simulink model "MEEN432_Project3_start"  (R2024b)
settings: Solver=VariableStepAuto  StartTime=0.0  StopTime=344  RelTol=1e-3
values from neighbouring files (symbols this model uses):
  eff = 0.9    [Project3_init.m]
  epa = urban_epa    [Project3_init.m]
  F_drag = 0    [Project3_init.m]
  G = 100    [Project3_init.m]
  I = 1600    [Project3_init.m]
  I_w = 0    [Project3_init.m]
  input_gear_inertia = 0.1    [Project3_init.m]
  m = 1000    [Project3_init.m]
  output_gear_inertia = 0.001    [Project3_init.m]
  r = 0.3    [Project3_init.m]
  tau_l = 1    [Project3_init.m]
  time = urban_time    [Project3_init.m]
  Tm_max = 350    [Project3_init.m]
libraries: slpidlib x1
settings Model: Creator=flare  LastModifiedBy=jpalm
settings RTWCC: GPUComputeCapability=3.5

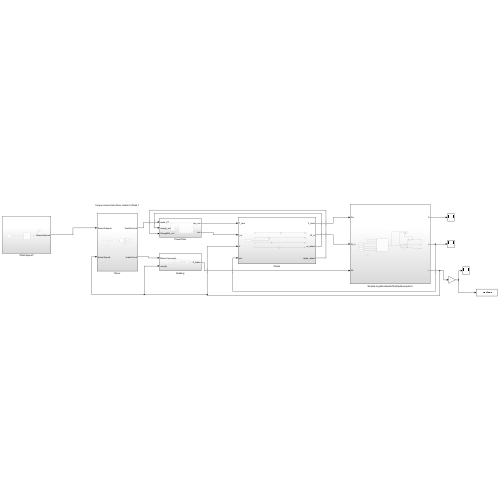
[thumbnail: Simulink's stored preview of the top-level diagram]
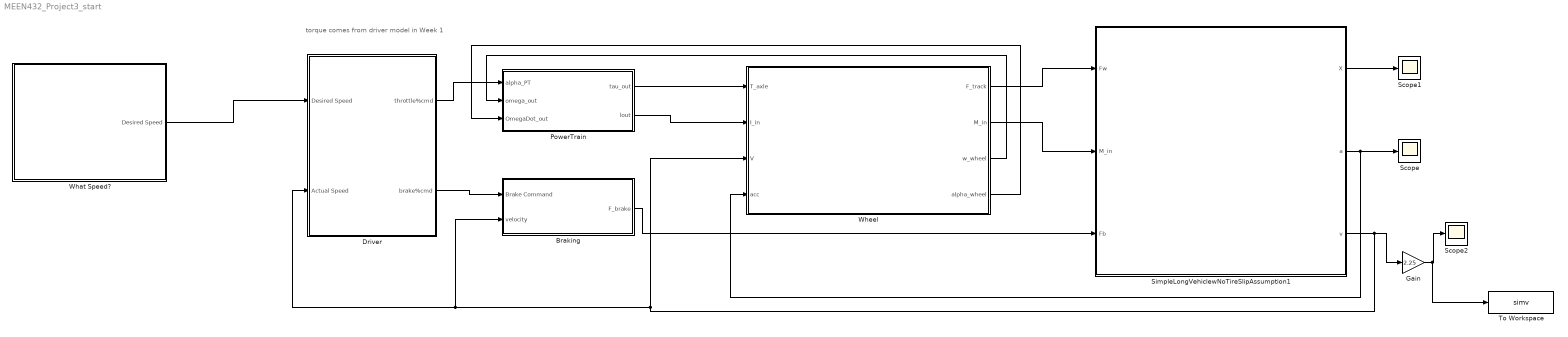
== system MEEN432_Project3_start ==
  note: torque comes from driver model in Week 1
  Braking : Subsystem
  Driver : Subsystem
  Gain : Gain  Gain=2.25
  PowerTrain : Subsystem
  Scope : Scope
  Scope1 : Scope
  Scope2 : Scope
  SimpleLongVehiclewNoTireSlipAssumption1 : Subsystem
  To Workspace : ToWorkspace  VariableName=simv  SaveFormat=Timeseries  SampleTime=-1
  What Speed? : Subsystem
  Wheel : Subsystem
  wires:
  What Speed?/1(Desired Speed) -> Driver/1(Desired Speed)
  SimpleLongVehiclewNoTireSlipAssumption1/3(v) -> Wheel/3(V), Braking/2(velocity), Driver/2(Actual Speed), Gain/1
  SimpleLongVehiclewNoTireSlipAssumption1/2(a) -> Scope/1, Wheel/4(acc)
  SimpleLongVehiclewNoTireSlipAssumption1/1(X) -> Scope1/1
  Driver/1(throttle%cmd) -> PowerTrain/1(alpha_PT)
  Driver/2(brake%cmd) -> Braking/1(Brake Command)
  PowerTrain/1(tau_out) -> Wheel/1(T_axle)
  Wheel/1(F_track) -> SimpleLongVehiclewNoTireSlipAssumption1/1(Fw)
  Wheel/2(M_in) -> SimpleLongVehiclewNoTireSlipAssumption1/2(M_in)
  Braking/1(F_brake) -> SimpleLongVehiclewNoTireSlipAssumption1/3(Fb)
  Gain/1 -> To Workspace/1, Scope2/1
  Wheel/3(w_wheel) -> PowerTrain/2(omega_out)
  Wheel/4(alpha_wheel) -> PowerTrain/3(OmegaDot_out)
  PowerTrain/2(lout) -> Wheel/2(I_in)

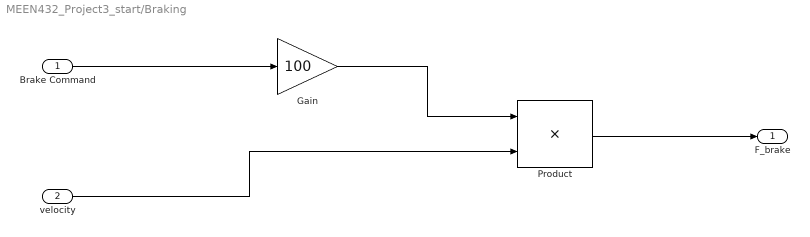
== system MEEN432_Project3_start/Braking ==
  Brake Command : Inport
  velocity : Inport  Port=2
  Gain : Gain  Gain=100
  Product : Product
  F_brake : Outport
  wires:
  Brake Command/1 -> Gain/1
  Gain/1 -> Product/1
  velocity/1 -> Product/2
  Product/1 -> F_brake/1

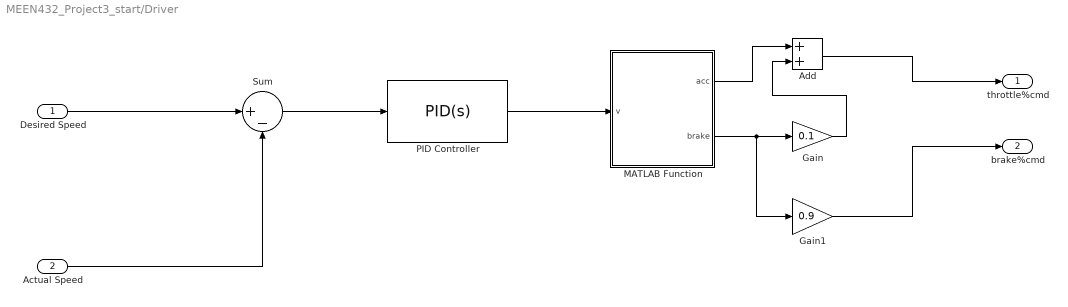
== system MEEN432_Project3_start/Driver ==
  Desired Speed : Inport
  Actual Speed : Inport  Port=2
  Add : Sum
  Gain : Gain  Gain=0.1
  Gain1 : Gain  Gain=0.9
  MATLAB Function : MATLAB Function  TreatAsAtomicUnit=on
  PID Controller : slpidlib/PID Controller  Controller=PID  Form=Parallel  TimeDomain=Continuous-time  UseExternalTs=off  SampleTime=-1  IntegratorMethod=Forward Euler  FilterMethod=Forward Euler  ControllerParametersSource=internal  P=1  I=1  UseKiTs=off  D=0  UseExternalDerivativeSource=off  N=100  UseFilter=on  TunerSelectOption=Transfer Function Based (PID Tuner App)  InitialConditionSource=internal  InitialConditionForIntegrator=0  InitialConditionForFilter=0  DifferentiatorICPrevScaledInput=0  ExternalReset=none  TrackingMode=off  Kt=1  LimitOutput=off  SatLimitsSource=internal  UpperSaturationLimit=inf  LowerSaturationLimit=-inf  LinearizeAsGain=on  AntiWindupMode=none  Kb=1  LimitIntegrator=off  UpperIntegratorSaturationLimit=inf  LowerIntegratorSaturationLimit=-inf  POutMin=[]  POutMax=[]  IOutMin=[]  IOutMax=[]  DOutMin=[]  DOutMax=[]  NOutMin=[]  NOutMax=[]  SumOutMin=[]  SumOutMax=[]  SaturationOutMin=[]  SaturationOutMax=[]  PParamMin=[]  PParamMax=[]  IParamMin=[]  IParamMax=[]  DParamMin=[]  DParamMax=[]  NParamMin=[]  NParamMax=[]  KbParamMin=[]  KbParamMax=[]  KtParamMin=[]  KtParamMax=[]  KbOutMin=[]  KbOutMax=[]  KtOutMin=[]  KtOutMax=[]  IntegratorOutMin=[]  IntegratorOutMax=[]  FilterOutMin=[]  FilterOutMax=[]  SumI1OutMin=[]  SumI1OutMax=[]  SumI2OutMin=[]  SumI2OutMax=[]  SumI3OutMin=[]  SumI3OutMax=[]  SumI4OutMin=[]  SumI4OutMax=[]  SumDOutMin=[]  SumDOutMax=[]  DifferentiatorOutMin=[]  DifferentiatorOutMax=[]  FilterDiffOutCoefMin=[]  FilterDiffOutCoefMax=[]  ReciprocalOutMin=[]  ReciprocalOutMax=[]  SumDenOutMin=[]  SumDenOutMax=[]  SumNumOutMin=[]  SumNumOutMax=[]  DivideOutMin=[]  DivideOutMax=[]  UdiffTsProdOutMin=[]  UdiffTsProdOutMax=[]  NTsProdOutMin=[]  NTsProdOutMax=[]  UintegralTsProdOutMin=[]  UintegralTsProdOutMax=[]  UngainTsProdOutMin=[]  UngainTsProdOutMax=[]  ClampingZeroOutDataTypeStr=Inherit: Inherit via back propagation  ClampingZeroOutMin=[]  ClampingZeroOutMax=[]  FilterDenConstantOutDataTypeStr=Inherit: Inherit via back propagation  FilterDenConstantOutMin=[]  FilterDenConstantOutMax=[]  PCopyOutDataTypeStr=Inherit: Inherit via back propagation  PCopyOutMin=[]  PCopyOutMax=[]  NCopyOutDataTypeStr=Inherit: Inherit via back propagation  NCopyOutMin=[]  NCopyOutMax=[]  IntegratorContinuousStateAttributes=''  IntegratorStateMustResolveToSignalObject=off  IntegratorRTWStateStorageClass=Auto  FilterContinuousStateAttributes=''  FilterStateMustResolveToSignalObject=off  FilterRTWStateStorageClass=Auto  ParallelPVariant=InternalParameters  IdealPVariant=Disabled  IVariant=InternalParameters  DVariant=InternalParameters  IntegratorVariant=Continuous  SatVariant=Disabled  AWVariant=Passthrough  PCopyVariant=Disabled  TRVariant=Disabled  FdbkBlocksVariant=Forward  IdealPFdbkVariant=Disabled  SatFdbkVariant=Disabled  DerivativeFilterVariant=ContFilter  NVariant=InternalParameters  NCopyVariant=Disabled  FilterICVariant=InternalICsFilter  IntegratorICVariant=InternalICs  ExternalResetVariant=Disabled  TRSumVariant=Passthrough  SumFdbkVariant=Disabled  SumVariant=Sum_PID  TsampFilterVariant=InternalTs  TsampNgainVariant=Passthrough  TsampIntegralVariant=Disabled_SignalSpec  ExternalSaturationOutDataTypeStr=Inherit: Same as second input  DerivativeSourceVariant=ErrorSignal  PreIntVariant=InternalPreInt
  Sum : Sum  Inputs=|+-
  throttle%cmd : Outport
  brake%cmd : Outport  Port=2
  wires:
  Actual Speed/1 -> Sum/2
  Sum/1 -> PID Controller/1
  PID Controller/1 -> MATLAB Function/1(v)
  MATLAB Function/1(acc) -> Add/1
  MATLAB Function/2(brake) -> Gain1/1, Gain/1
  Gain/1 -> Add/2
  Gain1/1 -> brake%cmd/1
  Add/1 -> throttle%cmd/1
  Desired Speed/1 -> Sum/1

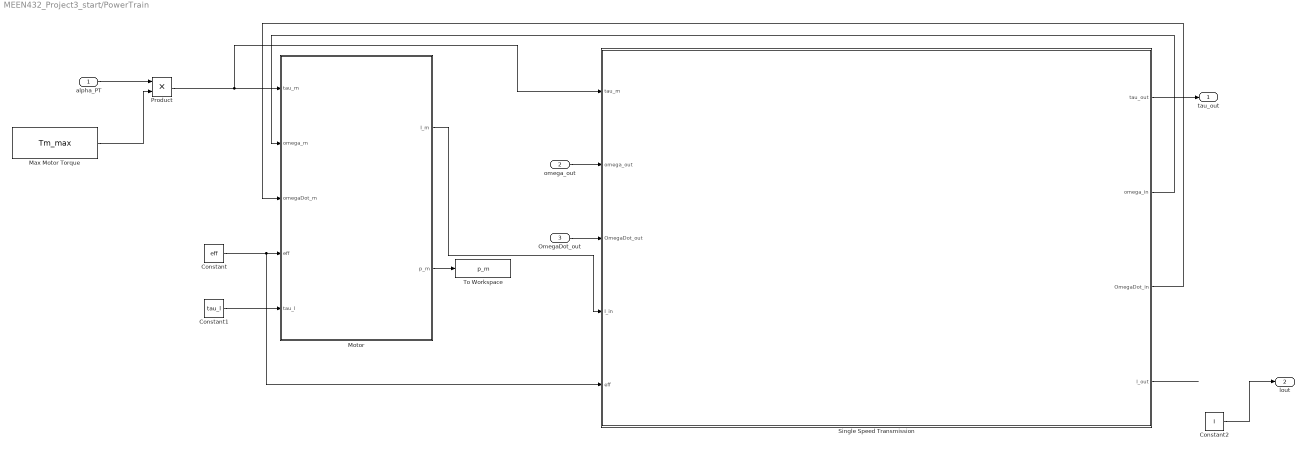
== system MEEN432_Project3_start/PowerTrain ==
  alpha_PT : Inport
  omega_out : Inport  Port=2
  OmegaDot_out : Inport  Port=3
  Constant : Constant  Value=eff
  Constant1 : Constant  Value=tau_l
  Constant2 : Constant  Value=I
  Max Motor Torque : Constant  Value=Tm_max
  Motor : MATLAB Function  TreatAsAtomicUnit=on
  Product : Product
  Single Speed Transmission : Subsystem
  To Workspace : ToWorkspace  VariableName=p_m  SaveFormat=Timeseries  SampleTime=-1
  tau_out : Outport
  lout : Outport  Port=2
  wires:
  alpha_PT/1 -> Product/1
  Max Motor Torque/1 -> Product/2
  omega_out/1 -> Single Speed Transmission/2(omega_out)
  OmegaDot_out/1 -> Single Speed Transmission/3(OmegaDot_out)
  Single Speed Transmission/1(tau_out) -> tau_out/1
  Single Speed Transmission/2(omega_in) -> Motor/2(omega_m)
  Single Speed Transmission/3(OmegaDot_in) -> Motor/3(omegaDot_m)
  Product/1 -> Single Speed Transmission/1(tau_m), Motor/1(tau_m)
  Motor/1(I_m) -> Single Speed Transmission/4(I_in)
  Motor/2(p_m) -> To Workspace/1
  Constant/1 -> Single Speed Transmission/5(eff), Motor/4(eff)
  Constant1/1 -> Motor/5(tau_l)
  Single Speed Transmission/4(l_out) -> ?
  Constant2/1 -> lout/1

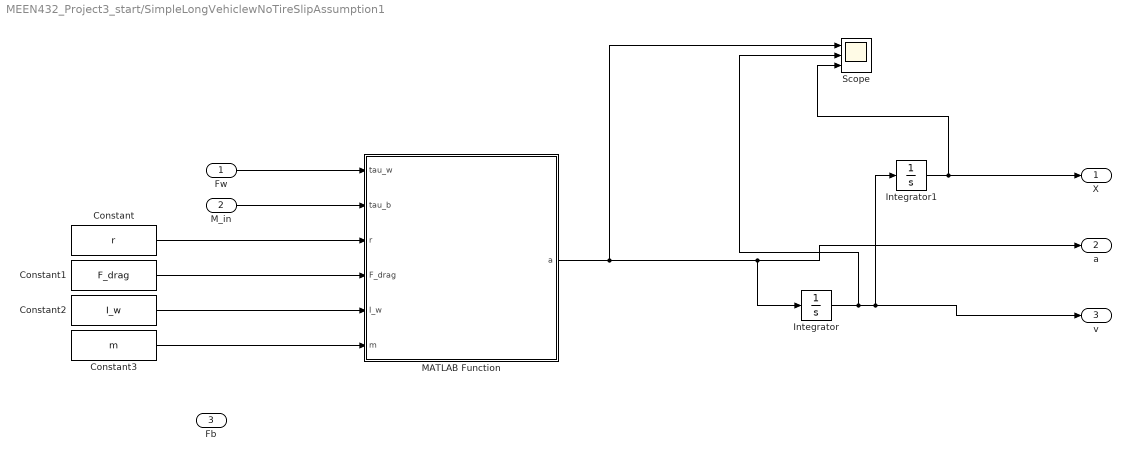
== system MEEN432_Project3_start/SimpleLongVehiclewNoTireSlipAssumption1 ==
  Fw : Inport
  M_in : Inport  Port=2
  Fb : Inport  Port=3
  Constant : Constant  Value=r
  Constant1 : Constant  Value=F_drag
  Constant2 : Constant  Value=I_w
  Constant3 : Constant  Value=m
  Integrator : Integrator
  Integrator1 : Integrator
  MATLAB Function : MATLAB Function  TreatAsAtomicUnit=on
  Scope : Scope  NumInputPorts=3
  X : Outport
  a : Outport  Port=2
  v : Outport  Port=3
  wires:
  MATLAB Function/1(a) -> Scope/1, Integrator/1, a/1
  Integrator/1 -> Scope/2, Integrator1/1, v/1
  Integrator1/1 -> Scope/3, X/1
  Fw/1 -> MATLAB Function/1(tau_w)
  M_in/1 -> MATLAB Function/2(tau_b)
  Constant/1 -> MATLAB Function/3(r)
  Constant1/1 -> MATLAB Function/4(F_drag)
  Constant2/1 -> MATLAB Function/5(I_w)
  Constant3/1 -> MATLAB Function/6(m)

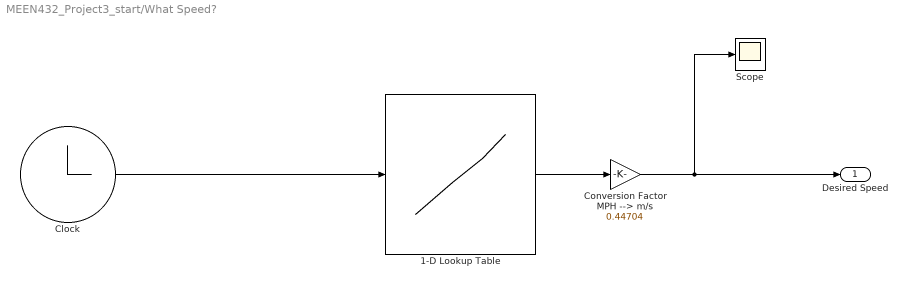
== system MEEN432_Project3_start/What Speed? ==
  1-D Lookup Table : Lookup_n-D  NumberOfTableDimensions=1  BreakpointsForDimension1=time  Table=epa  InternalRulePriority=Speed  RndMeth=Simplest
  Clock : Clock
  Conversion Factor MPH --> m/s : Gain  Gain=0.44704
  Scope : Scope
  Desired Speed : Outport
  wires:
  Clock/1 -> 1-D Lookup Table/1
  1-D Lookup Table/1 -> Conversion Factor MPH --> m/s/1
  Conversion Factor MPH --> m/s/1 -> Scope/1, Desired Speed/1

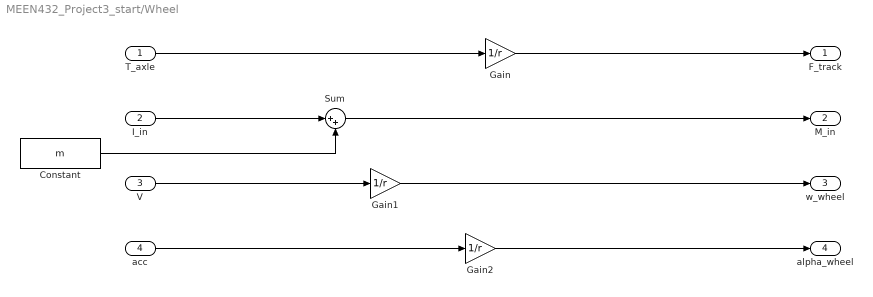
== system MEEN432_Project3_start/Wheel ==
  T_axle : Inport
  I_in : Inport  Port=2
  V : Inport  Port=3
  acc : Inport  Port=4
  Constant : Constant  Value=m
  Gain : Gain  Gain=1/r
  Gain1 : Gain  Gain=1/r
  Gain2 : Gain  Gain=1/r
  Sum : Sum  Inputs=|++
  F_track : Outport
  M_in : Outport  Port=2
  w_wheel : Outport  Port=3
  alpha_wheel : Outport  Port=4
  wires:
  T_axle/1 -> Gain/1
  Gain/1 -> F_track/1
  I_in/1 -> Sum/1
  Sum/1 -> M_in/1
  Constant/1 -> Sum/2
  V/1 -> Gain1/1
  Gain1/1 -> w_wheel/1
  acc/1 -> Gain2/1
  Gain2/1 -> alpha_wheel/1

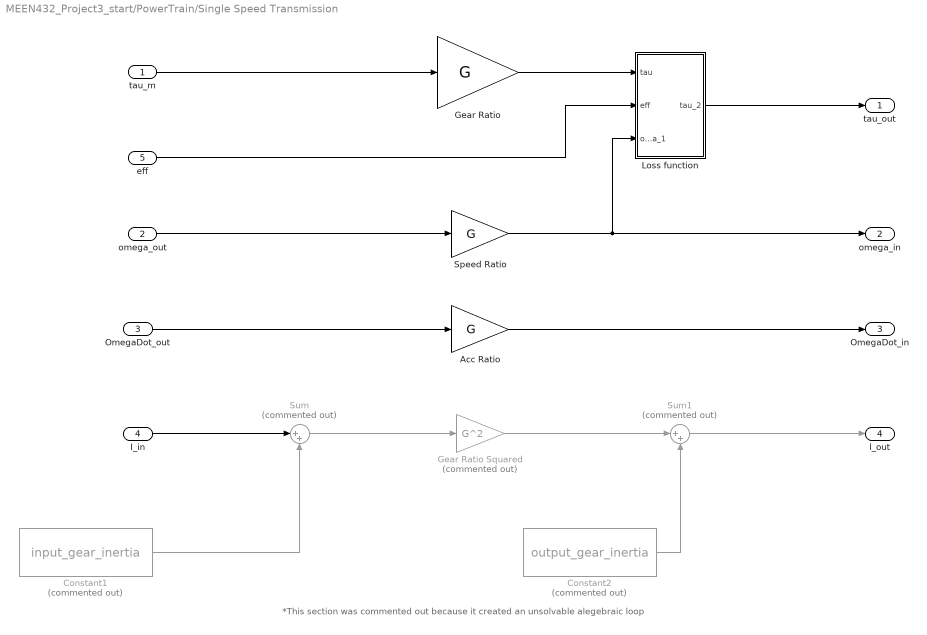
== system MEEN432_Project3_start/PowerTrain/Single Speed Transmission ==
  note: *This section was commented out because it created an unsolvable alegebraic loop
  tau_m : Inport
  omega_out : Inport  Port=2
  OmegaDot_out : Inport  Port=3
  I_in : Inport  Port=4
  eff : Inport  Port=5
  Acc Ratio : Gain  Gain=G
  Constant1 : Constant  Commented=on  Value=input_gear_inertia
  Constant2 : Constant  Commented=on  Value=output_gear_inertia
  Gear Ratio : Gain  Gain=G
  Gear Ratio Squared : Gain  Commented=on  Gain=G^2
  Loss function : MATLAB Function  TreatAsAtomicUnit=on
  Speed Ratio : Gain  Gain=G
  Sum : Sum  Commented=on  Inputs=|++
  Sum1 : Sum  Commented=on  Inputs=|++
  tau_out : Outport
  omega_in : Outport  Port=2
  OmegaDot_in : Outport  Port=3
  l_out : Outport  Port=4
  wires:
  Speed Ratio/1 -> omega_in/1, Loss function/3(omega_1)
  tau_m/1 -> Gear Ratio/1
  Acc Ratio/1 -> OmegaDot_in/1
  Loss function/1(tau_2) -> tau_out/1
  Gear Ratio/1 -> Loss function/1(tau)
  omega_out/1 -> Speed Ratio/1
  OmegaDot_out/1 -> Acc Ratio/1
  eff/1 -> Loss function/2(eff)
  I_in/1 -> Sum/1
  Sum/1 -> Gear Ratio Squared/1
  Constant1/1 -> Sum/2
  Gear Ratio Squared/1 -> Sum1/1
  Sum1/1 -> l_out/1
  Constant2/1 -> Sum1/2

== matlab function MEEN432_Project3_start/PowerTrain/Motor ==
  data: tau_m input; omega_m input; omegaDot_m input; I_m output; p_m output; eff input; tau_l input
function [I_m, p_m]= fcn(tau_m, omega_m, omegaDot_m, eff, tau_l)

I_m = (tau_m - tau_l)/omegaDot_m;
p_m = tau_m*omega_m*eff^(sign(tau_m*omega_m));

== matlab function MEEN432_Project3_start/PowerTrain/Single Speed Transmission/Loss function ==
  data: tau input; eff input; tau_2 output; omega_1 input
function tau_2 = fcn(tau, eff, omega_1)

tau_2 = tau*eff^sign(tau*omega_1);

== matlab function MEEN432_Project3_start/Driver/MATLAB Function ==
  data: v input; acc output; brake output
function [acc, brake] = fcn(v)

if v > 0
    acc = v;
    brake = 0;
elseif v < 0
    acc = 0;
    brake = v;
else
    acc = 0;
    brake = 0;
end

== matlab function MEEN432_Project3_start/SimpleLongVehiclewNoTireSlipAssumption1/MATLAB Function ==
  data: tau_w input; a output; tau_b input; r input; F_drag input; I_w input; m input
function a = fcn(tau_w, tau_b, r, F_drag, I_w, m)
theta = 90; % degrees
g = 9.81; % m/s^2

num = ((tau_w - tau_b) / r) - F_drag;
a = num / ((I_w / r^2) + m);
